simulink model "pwr_amp_1"  (Simulink 7.4)
settings: Solver=ode45  StartTime=0.0  StopTime=inf  MaxStep=1/(10*1e6)  RelTol=1e-3  AbsTol=1e-3
PreLoadFcn:
  | bessel_1
values from neighbouring files (symbols this model uses):
  C3 = c3/(R*w)    (= 1.52191914332e-07)    [bessel_1.m]
  L2 = l2*R/w    (= 1.55653534344e-05)    [bessel_1.m]
  L4 = l4*R/w    (= 3.35816929924e-06)    [bessel_1.m]
undefined symbols (not defined in the file or in its folder): C1
libraries: powerlib x13, simulink x3, simpower_extensions_1 x1, simulink_extras x1
settings Model: Creator=dbenson  LastModifiedBy=Dick
settings SolverCC: ZeroCrossControl=EnableAll
settings DataIOCC: LimitDataPoints=off  SaveOutput=off  SaveTime=off  SignalLoggingName=sigsOut
settings OptimizationCC: BooleanDataType=off  InlineInvariantSignals=on  InitFltsAndDblsToZero=on
settings DebuggingCC: SaveWithParameterizedLinksMsg=none  SignalResolutionControl=TryResolveAllWithWarning  SolverPrmCheckMsg=none  MultiTaskDSMMsg=warning  MultiTaskCondExecSysMsg=none  StrictBusMsg=None
settings HardwareCC: TargetUnknown=on
settings RTWCC: IncludeERTFirstTime=on
settings GRTTargetCC: TargetFcnLib=ansi_tfl_tmw.mat

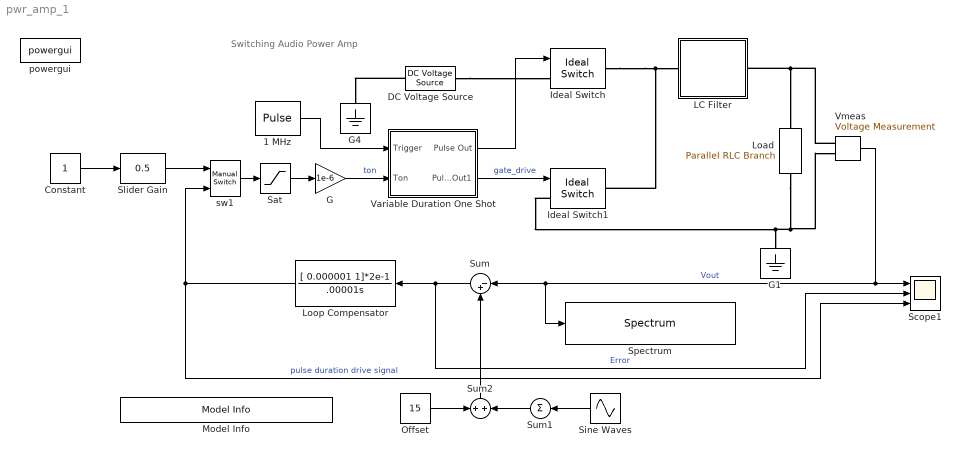
== system pwr_amp_1 ==
  note: Switching Audio Power Amp
  1 MHz : DiscretePulseGenerator  PulseType=Time based  Amplitude=1  Period=1/1e6;  PulseWidth=50  PhaseDelay=.5e-6  SampleTime=1
  Constant : Constant  OutDataType=sfix(16)  OutScaling=2^0
  DC Voltage Source : powerlib/Electrical Sources/DC Voltage Source  Description=source block  DialogController=POWERSYS.PowerSysDialog  SystemSampleTime=-1  Amplitude=30  Measurements=None
      settings: AttributesFormatString=\n
  G : Gain  Gain=1e-6  ParameterDataType=sfix(16)  ParameterScaling=2^0  OutDataType=sfix(16)  OutScaling=2^0  SaturateOnIntegerOverflow=on  OutDataTypeStr=Inherit: Same as input  ParamDataTypeStr=Inherit: Same as input
  G1 : powerlib/Elements/Ground  DialogController=POWERSYS.PowerSysDialog  PhysicalDomain=powersysdomain  SubClassName=unknown  LeftPortType=p1  RightPortType=p1  LConnTagsString=a
  G4 : powerlib/Elements/Ground  DialogController=POWERSYS.PowerSysDialog  PhysicalDomain=powersysdomain  SubClassName=unknown  LeftPortType=p1  RightPortType=p1  LConnTagsString=a
  Ideal Switch : powerlib/Power Electronics/Ideal Switch  DialogController=POWERSYS.PowerSysDialog  SystemSampleTime=-1  Ron=0.1  Lon=0  IC=0  Rs=0  Cs=0  Measurements=off
      settings: AttributesFormatString=\n
  Ideal Switch1 : powerlib/Power Electronics/Ideal Switch  DialogController=POWERSYS.PowerSysDialog  SystemSampleTime=-1  Ron=0.1  Lon=0  IC=0  Rs=0  Cs=0  Measurements=off
      settings: AttributesFormatString=\n
  LC Filter : Subsystem
  Load : powerlib/Elements/Parallel RLC Branch  DialogController=POWERSYS.PowerSysDialog  PhysicalDomain=powersysdomain  SubClassName=unknown  LeftPortType=p1  RightPortType=p1  LConnTagsString=a  RConnTagsString=__new0  BranchType=R  Resistance=8  Inductance=1.0  SetiL0=off  InitialCurrent=0  Capacitance=1.0  Setx0=off  InitialVoltage=0  Measurements=None
  Loop Compensator : TransferFcn  Numerator=[ 0.000001 1]*2e-1  Denominator=[.00001 0]
  Model Info : simulink/Model-Wide Utilities/Model Info  SystemSampleTime=-1  InitialBlockCM=None  BlockCM=None  Frame=on  DisplayStringWithTags=Copywrite 2005-2010 The MathWorks, Inc.  HorizontalTextAlignment=Center  LeftAlignmentValue=0.5  SourceBlockDiagram=pwr_amp_1  TagMaxNumber=20
  Offset : Constant  Value=15  OutDataType=sfix(16)  OutScaling=2^0
  Sat : Saturate  UpperLimit=0.95  LowerLimit=.01
  Scope1 : Scope  NumInputPorts=3
      settings: TimeRange=0.01  YMin=0~-15~0.1  YMax=30~20~0.9  SaveName=ScopeData2
  Sine Waves : Sin  Amplitude=5  Bias=0  Frequency=2*pi*[2000,2500]  Phase=0  Samples=10  SampleTime=0  Offset=0
  Slider Gain : simulink/Math Operations/Slider Gain  SystemSampleTime=-1  low=0  gain=0.5  high=1
  Spectrum : simpower_extensions_1/Spectrum  Description=Spectrum Analyzer  SystemSampleTime=-1  BW=20e3  Zo=8
  Sum : Sum  Inputs=|-+  OutDataType=sfix(16)  OutScaling=2^0  SaturateOnIntegerOverflow=on  InputSameDT=on  OutDataTypeStr=Inherit: Same as first input
  Sum1 : Sum  Inputs=+  OutDataType=sfix(16)  OutScaling=2^0
  Sum2 : Sum  OutDataType=sfix(16)  OutScaling=2^0
  Variable Duration One Shot : Subsystem
  Vmeas : powerlib/Measurements/Voltage Measurement  Tag=PoWeRsYsTeMmEaSuReMeNt  DialogController=POWERSYS.PowerSysDialog  SystemSampleTime=-1  PhasorSimulation=off  OutputType=Magnitude  PSBequivalent=0
  powergui : powerlib/powergui  SystemSampleTime=-1  SimulationMode=Continuous  SampleTime=50e-6  frequency=60  SPID=off  DisableSnubberDevices=off  DisableRonSwitches=off  DisableVfSwitches=off  SwTol=0  Interpol=off  frequencyindice=0  echomessages=off  HookPort=off  DisplayEquations=off  FunctionMessages=off  EnableUseOfTLC=off  x0status=blocks  RestoreLinks=warning  Frange=[0:2:500]  Ylog=off  Xlog=on  ShowGrid=off  save=off  variable=ZData  ZoomFFT=on  StartTime=0.0  cycles=1  DisplayStyle=1  fundamental=60  FreqAxis=off  MaxFrequency=1000  frequencyindicesteady=1  RmsSteady=1  display=off  Ts=0  methode=off
  sw1 : simulink/Signal Routing/Manual Switch  SystemSampleTime=-1  sw=0  action=0  varsize=off
  wires:
  1 MHz/1 -> Variable Duration One Shot/1(Trigger)
  Loop Compensator/1 -> sw1/2, Scope1/3  "pulse duration drive signal"
  Sum/1 -> Scope1/2, Loop Compensator/1  "Error"
  G/1 -> Variable Duration One Shot/2(Ton)  "ton"
  Sat/1 -> G/1
  Vmeas/1 -> Scope1/1, Sum/1, Spectrum/1  "Vout"
  Variable Duration One Shot/1(Pulse Out) -> Ideal Switch/1
  Variable Duration One Shot/2(Pulse Out1) -> Ideal Switch1/1  "gate_drive"
  sw1/1 -> Sat/1
  Constant/1 -> Slider Gain/1
  Slider Gain/1 -> sw1/1
  Sine Waves/1 -> Sum1/1
  Sum1/1 -> Sum2/2
  Sum2/1 -> Sum/2
  Offset/1 -> Sum2/1
  connections:
  DC Voltage Source/RConn1 -- Ideal Switch/LConn1
  Ideal Switch/RConn1 -- Ideal Switch1/RConn1 -- LC Filter/LConn1
  Load/RConn1 -- Ideal Switch1/LConn1 -- G1/LConn1 -- Vmeas/LConn2
  DC Voltage Source/LConn1 -- G4/LConn1
  Vmeas/LConn1 -- LC Filter/RConn1 -- Load/LConn1

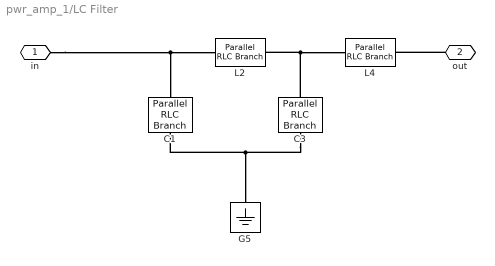
== system pwr_amp_1/LC Filter ==
  C1 : powerlib/Elements/Parallel RLC Branch  DialogController=POWERSYS.PowerSysDialog  PhysicalDomain=powersysdomain  SubClassName=unknown  LeftPortType=p1  RightPortType=p1  LConnTagsString=a  RConnTagsString=__new0  BranchType=C  Resistance=1.0  Inductance=1.0  SetiL0=off  InitialCurrent=0  Capacitance=C1  Setx0=off  InitialVoltage=0  Measurements=None
  C3 : powerlib/Elements/Parallel RLC Branch  DialogController=POWERSYS.PowerSysDialog  PhysicalDomain=powersysdomain  SubClassName=unknown  LeftPortType=p1  RightPortType=p1  LConnTagsString=a  RConnTagsString=__new0  BranchType=C  Resistance=1.0  Inductance=1.0  SetiL0=off  InitialCurrent=0  Capacitance=C3  Setx0=off  InitialVoltage=0  Measurements=None
  G5 : powerlib/Elements/Ground  DialogController=POWERSYS.PowerSysDialog  PhysicalDomain=powersysdomain  SubClassName=unknown  LeftPortType=p1  RightPortType=p1  LConnTagsString=a
  L2 : powerlib/Elements/Parallel RLC Branch  DialogController=POWERSYS.PowerSysDialog  PhysicalDomain=powersysdomain  SubClassName=unknown  LeftPortType=p1  RightPortType=p1  LConnTagsString=a  RConnTagsString=__new0  BranchType=L  Resistance=1.0  Inductance=L2  SetiL0=off  InitialCurrent=0  Capacitance=1.0  Setx0=off  InitialVoltage=0  Measurements=None
  L4 : powerlib/Elements/Parallel RLC Branch  DialogController=POWERSYS.PowerSysDialog  PhysicalDomain=powersysdomain  SubClassName=unknown  LeftPortType=p1  RightPortType=p1  LConnTagsString=a  RConnTagsString=__new0  BranchType=L  Resistance=1.0  Inductance=L4  SetiL0=off  InitialCurrent=0  Capacitance=1.0  Setx0=off  InitialVoltage=0  Measurements=None
  in : PMIOPort  Port=1  Side=Left
  out : PMIOPort  Port=2  Side=Right
  connections:
  C3/LConn1 -- C1/LConn1 -- G5/LConn1
  C3/RConn1 -- L2/RConn1 -- L4/LConn1
  out/RConn1 -- L4/RConn1
  in/RConn1 -- C1/RConn1 -- L2/LConn1

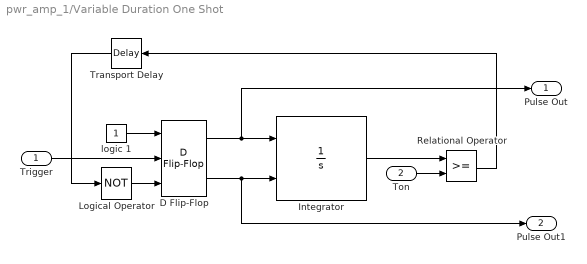
== system pwr_amp_1/Variable Duration One Shot ==
  Trigger : Inport  OutDataType=sfix(16)  OutScaling=2^0
  Ton : Inport  Port=2  OutDataType=sfix(16)  OutScaling=2^0
  D Flip-Flop : simulink_extras/Flip Flops/D Flip-Flop  SystemSampleTime=-1
  Integrator : Integrator  ExternalReset=level
  Logical Operator : Logic  Operator=NOT
  Relational Operator : RelationalOperator  InputSameDT=on
  Transport Delay : TransportDelay  DelayTime=10e-9
  logic 1 : Constant  OutDataType=sfix(16)  OutScaling=2^0
  Pulse Out : Outport  OutDataType=sfix(16)  OutScaling=2^0
  Pulse Out1 : Outport  Port=2  OutDataType=sfix(16)  OutScaling=2^0
  wires:
  D Flip-Flop/2 -> Integrator/2, Pulse Out1/1
  logic 1/1 -> D Flip-Flop/1
  Relational Operator/1 -> Transport Delay/1
  Logical Operator/1 -> D Flip-Flop/3
  Integrator/1 -> Relational Operator/1
  D Flip-Flop/1 -> Integrator/1, Pulse Out/1
  Trigger/1 -> D Flip-Flop/2
  Ton/1 -> Relational Operator/2
  Transport Delay/1 -> Logical Operator/1
